simulink library "csc_sta_star_tracker_lib"  (R2014b)
settings: Solver=ode45  SolverMode=SingleTasking  StartTime=0.0  StopTime=10.0  RelTol=1e-3
values from neighbouring files (symbols this model uses):
  sta_body_to_head1 = rot_angles_to_quat([ sta_body_to_head1_rotz sta_body_to_head1_roty sta_body_to_head1_rotx] )    [csc_sta_star_tracker_prep.m]
undefined symbols (not defined in the file or in its folder): pwr_sta_on_state
libraries: util_common_lib x5, util_info_lib x2, simulink x1, csc_mir_miru_lib x1, csu_dmo_dtu_message_output_lib x1, csu_trh_tracker_head_lib x1
settings Model: Creator=eleanor  LastModifiedBy=mstewart

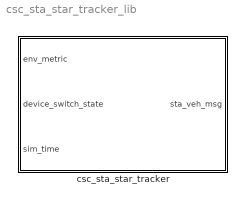
== system csc_sta_star_tracker_lib ==
  csc_sta_star_tracker : Subsystem  SystemSampleTime=0.1

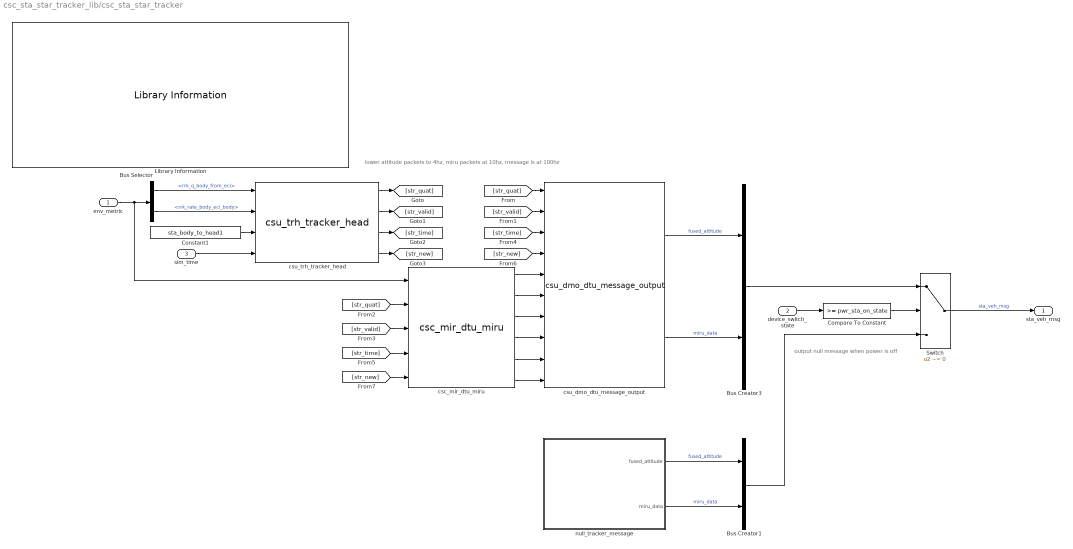
== system csc_sta_star_tracker_lib/csc_sta_star_tracker ==
  note: lower attitude packets to 4hz, miru packets at 10hz, message is at 100hz
  note: output null message when power is off
  env_metric : Inport
  device_switch_state : Inport  Port=2
  sim_time : Inport  Port=3
  Bus Creator1 : BusCreator  Inputs=2
  Bus Creator3 : BusCreator  Inputs=2
  Bus Selector : BusSelector  OutputSignals=lander_state_bus.rrk_q_body_from_eci,lander_state_bus.rrk_rate_body_eci_body
  Compare To Constant : simulink/Logic and Bit Operations/Compare To Constant  relop=>=  const=pwr_sta_on_state  OutDataTypeStr=boolean
  Constant1 : Constant  Value=sta_body_to_head1
  Library Information : util_info_lib/Library Information  owner='NONE'
  Switch : Switch  Criteria=u2 ~= 0
  csc_mir_dtu_miru : csc_mir_miru_lib/csc_mir_dtu_miru
  csu_dmo_dtu_message_output : csu_dmo_dtu_message_output_lib/csu_dmo_dtu_message_output
  csu_trh_tracker_head : csu_trh_tracker_head_lib/csu_trh_tracker_head
  null_tracker_message : Subsystem
  sta_veh_msg : Outport
  wires:
  Compare To Constant/1 -> Switch/2
  device_switch_state/1 -> Compare To Constant/1
  Bus Selector/2 -> csu_trh_tracker_head/2  "<rrk_rate_body_eci_body>"
  env_metric/1 -> csc_mir_dtu_miru/1, Bus Selector/1
  Bus Selector/1 -> csu_trh_tracker_head/1  "<rrk_q_body_from_eci>"
  Switch/1 -> sta_veh_msg/1  "sta_veh_msg"
  Constant1/1 -> csu_trh_tracker_head/3
  csc_mir_dtu_miru/1 -> csu_dmo_dtu_message_output/5
  csc_mir_dtu_miru/2 -> csu_dmo_dtu_message_output/6
  csc_mir_dtu_miru/6 -> csu_dmo_dtu_message_output/10
  csc_mir_dtu_miru/5 -> csu_dmo_dtu_message_output/9
  csc_mir_dtu_miru/3 -> csu_dmo_dtu_message_output/7
  csc_mir_dtu_miru/4 -> csu_dmo_dtu_message_output/8
  csu_dmo_dtu_message_output/1 -> Bus Creator3/1  "fused_attitude"
  csu_dmo_dtu_message_output/2 -> Bus Creator3/2  "miru_data"
  Bus Creator3/1 -> Switch/1
  csu_trh_tracker_head/2 -> [str_valid]
  csu_trh_tracker_head/1 -> [str_quat]
  [str_valid] -> csu_dmo_dtu_message_output/2
  [str_quat] -> csu_dmo_dtu_message_output/1
  [str_valid] -> csc_mir_dtu_miru/3
  [str_quat] -> csc_mir_dtu_miru/2
  csu_trh_tracker_head/3 -> [str_time]
  [str_time] -> csu_dmo_dtu_message_output/3
  [str_time] -> csc_mir_dtu_miru/4
  csu_trh_tracker_head/4 -> [str_new]
  [str_new] -> csu_dmo_dtu_message_output/4
  [str_new] -> csc_mir_dtu_miru/5
  null_tracker_message/1(fused_attitude) -> Bus Creator1/1  "fused_attitude"
  null_tracker_message/2(miru_data) -> Bus Creator1/2  "miru_data"
  Bus Creator1/1 -> Switch/3
  sim_time/1 -> csu_trh_tracker_head/4

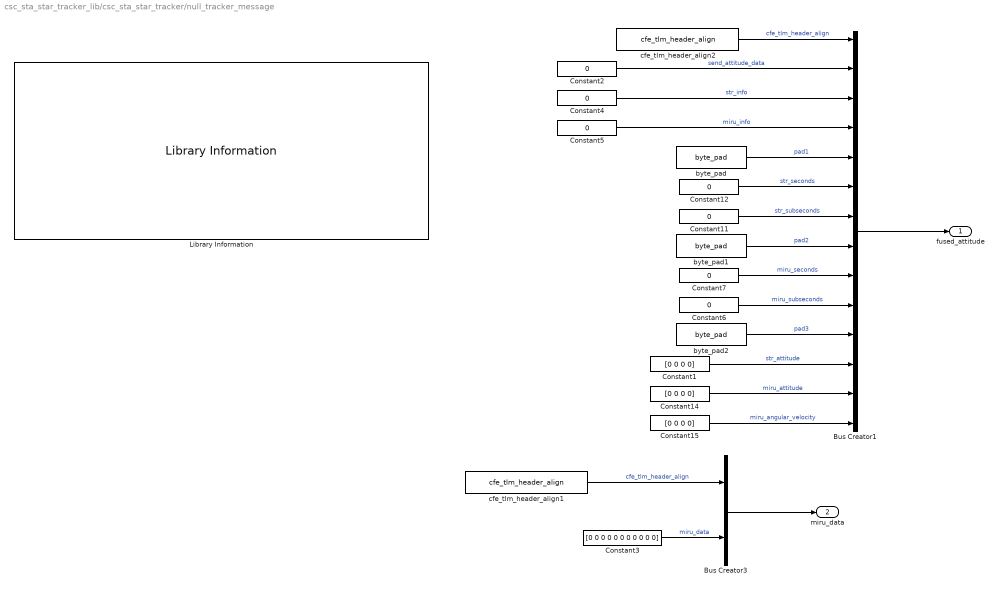
== system csc_sta_star_tracker_lib/csc_sta_star_tracker/null_tracker_message ==
  Bus Creator1 : BusCreator  Inputs=14  OutDataTypeStr=Bus: fused_attitude_msg  NonVirtualBus=on
  Bus Creator3 : BusCreator  Inputs=2  OutDataTypeStr=Bus: miru_data_msg  NonVirtualBus=on
  Constant1 : Constant  Value=[0 0 0 0]  OutDataTypeStr=int32
  Constant11 : Constant  Value=0  OutDataTypeStr=uint16
  Constant12 : Constant  Value=0  OutDataTypeStr=uint32
  Constant14 : Constant  Value=[0 0 0 0]  OutDataTypeStr=int32
  Constant15 : Constant  Value=[0 0 0 0]  OutDataTypeStr=int32
  Constant2 : Constant  Value=0  OutDataTypeStr=uint8
  Constant3 : Constant  Value=[0 0 0 0 0 0 0 0 0 0 0]  OutDataTypeStr=int16
  Constant4 : Constant  Value=0  OutDataTypeStr=uint8
  Constant5 : Constant  Value=0  OutDataTypeStr=uint8
  Constant6 : Constant  Value=0  OutDataTypeStr=uint16
  Constant7 : Constant  Value=0  OutDataTypeStr=uint32
  Library Information : util_info_lib/Library Information  owner='escrane'
  byte_pad : util_common_lib/byte_pad  n_bytes=1
  byte_pad1 : util_common_lib/byte_pad  n_bytes=2
  byte_pad2 : util_common_lib/byte_pad  n_bytes=2
  cfe_tlm_header_align1 : util_common_lib/cfe_tlm_header_align
  cfe_tlm_header_align2 : util_common_lib/cfe_tlm_header_align
  fused_attitude : Outport
  miru_data : Outport  Port=2
  wires:
  Bus Creator1/1 -> fused_attitude/1
  Constant15/1 -> Bus Creator1/14  "miru_angular_velocity"
  Constant14/1 -> Bus Creator1/13  "miru_attitude"
  Constant1/1 -> Bus Creator1/12  "str_attitude"
  byte_pad2/1 -> Bus Creator1/11  "pad3"
  byte_pad1/1 -> Bus Creator1/8  "pad2"
  byte_pad/1 -> Bus Creator1/5  "pad1"
  Constant5/1 -> Bus Creator1/4  "miru_info"
  Constant12/1 -> Bus Creator1/6  "str_seconds"
  Constant4/1 -> Bus Creator1/3  "str_info"
  Constant2/1 -> Bus Creator1/2  "send_attitude_data"
  cfe_tlm_header_align2/1 -> Bus Creator1/1  "cfe_tlm_header_align"
  Constant11/1 -> Bus Creator1/7  "str_subseconds"
  Constant7/1 -> Bus Creator1/9  "miru_seconds"
  Constant6/1 -> Bus Creator1/10  "miru_subseconds"
  cfe_tlm_header_align1/1 -> Bus Creator3/1  "cfe_tlm_header_align"
  Constant3/1 -> Bus Creator3/2  "miru_data"
  Bus Creator3/1 -> miru_data/1
